simulink model "objectDetector"  (R2016b)
settings: Solver=FixedStepAuto  StartTime=0.0  StopTime=inf  RelTol=1e-3
model workspace (MAT data in the model file):
  SL_ROS_VariableLengthArrays_MaxSizes.CommonInfo.ArrayTruncateAction = 'EmitWarning'
  SL_ROS_VariableLengthArrays_MaxSizes.MsgTypeMap = containers.Map
  SL_ROS_VariableLengthArrays_MaxSizes.MsgTypeMap.serialization.keys = {'sensor_msgs/LaserScan'}
  SL_ROS_VariableLengthArrays_MaxSizes.MsgTypeMap.serialization.values{1}(1).PropertyName = 'Ranges'
  SL_ROS_VariableLengthArrays_MaxSizes.MsgTypeMap.serialization.values{1}(1).DataType = 'single'
  SL_ROS_VariableLengthArrays_MaxSizes.MsgTypeMap.serialization.values{1}(1).MaxLength = 180
  SL_ROS_VariableLengthArrays_MaxSizes.MsgTypeMap.serialization.values{1}(2).PropertyName = 'Intensities'
  SL_ROS_VariableLengthArrays_MaxSizes.MsgTypeMap.serialization.values{1}(2).DataType = 'single'
  SL_ROS_VariableLengthArrays_MaxSizes.MsgTypeMap.serialization.values{1}(2).MaxLength = 128
  SL_ROS_VariableLengthArrays_MaxSizes.MsgTypeMap.serialization.uniformity = 0
  SL_ROS_VariableLengthArrays_MaxSizes.MsgTypeMap.serialization.keyType = 'char'
  SL_ROS_VariableLengthArrays_MaxSizes.MsgTypeMap.serialization.valueType = 'any'
undefined symbols (not defined in the file): Header
libraries: robotlib x4
settings Model: Creator=jupan  LastModifiedBy=fred
settings SolverCC: AutoInsertRateTranBlk=on
settings OptimizationCC: MaxStackSize=64
settings DebuggingCC: ParameterTunabilityLossMsg=error
settings HardwareCC: ProdBitPerPointer=32  ProdBitPerSizeT=32  ProdBitPerPtrDiffT=32  ProdLargestAtomicFloat=None  ProdIntDivRoundTo=Undefined  ProdEndianess=Unspecified  ProdWordSize=32  ProdHWDeviceType=Generic->Unspecified (assume 32-bit Generic)
settings RTWCC: SystemTargetFile=ert.tlc  HardwareBoard=Robot Operating System (ROS)  TLCOptions="-aInlineSetEventsForThisBaseRateFcn=TLC_FALSE -aSuppressMultiTaskScheduler=TLC_FALSE  -aRateBasedStepFcn=0"  TemplateMakefile=ert_default_tmf  Description=Embedded Coder  GenerateReport=on  Toolchain=Catkin  IncludeHyperlinkInReport=on  LaunchReport=on  TargetLang=C++  GenerateTraceInfo=on  GenerateTraceReport=on  GenerateTraceReportSl=on  GenerateTraceReportSf=on  GenerateTraceReportEml=on
settings CodeAppCC: ForceParamTrailComments=on  IgnoreCustomStorageClasses=off  OperatorAnnotations=on  SimulinkDataObjDesc=on  SFDataObjDesc=on  MATLABFcnDesc=on  InsertBlockDesc=on  MATLABSourceComments=on
settings ERTTargetCC: SupportVariableSizeSignals=on

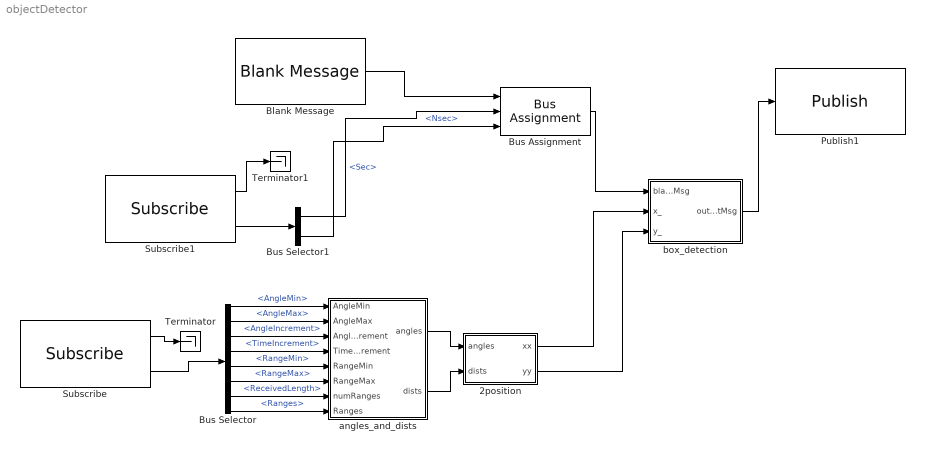
== system objectDetector ==
  " 2position" : MATLAB Function  TreatAsAtomicUnit=on
  Blank Message : robotlib/Blank Message  SourceLibraryInfo=This block requires Robotics System Toolbox  messageType=geometry_msgs/PolygonStamped  SampleTime=inf
  Bus Assignment : BusAssignment  AssignedSignals=Header.Stamp.Sec,Header.Stamp.Nsec
  Bus Selector : BusSelector  OutputSignals=AngleMin,AngleMax,AngleIncrement,TimeIncrement,RangeMin,RangeMax,Ranges_SL_Info.ReceivedLength,Ranges
  Bus Selector1 : BusSelector  OutputSignals=Clock_.Sec,Clock_.Nsec
  Publish1 : robotlib/Publish  SourceLibraryInfo=This block requires Robotics System Toolbox  topicSource=Specify your own  topic=/detections  messageType=geometry_msgs/PolygonStamped  messageQueueLength=1
  Subscribe : robotlib/Subscribe  SourceLibraryInfo=This block requires Robotics System Toolbox  topicSource=Select from ROS network  topic=/catvehicle/front_laser_points  messageType=sensor_msgs/LaserScan  sampleTime=-1  messageQueueLength=1
  Subscribe1 : robotlib/Subscribe  SourceLibraryInfo=This block requires Robotics System Toolbox  topicSource=Select from ROS network  topic=/clock  messageType=rosgraph_msgs/Clock  sampleTime=-1  messageQueueLength=1
  Terminator : Terminator
  Terminator1 : Terminator
  angles_and_dists : MATLAB Function  TreatAsAtomicUnit=on
  box_detection : MATLAB Function  TreatAsAtomicUnit=on
  wires:
  Subscribe/1 -> Terminator/1
  Subscribe/2 -> Bus Selector/1
  Bus Selector/1 -> angles_and_dists/1(AngleMin)  "<AngleMin>"
  Bus Selector/2 -> angles_and_dists/2(AngleMax)  "<AngleMax>"
  Bus Selector/3 -> angles_and_dists/3(AngleIncrement)  "<AngleIncrement>"
  Bus Selector/4 -> angles_and_dists/4(TimeIncrement)  "<TimeIncrement>"
  Bus Selector/5 -> angles_and_dists/5(RangeMin)  "<RangeMin>"
  Bus Selector/6 -> angles_and_dists/6(RangeMax)  "<RangeMax>"
  Bus Selector/7 -> angles_and_dists/7(numRanges)  "<ReceivedLength>"
  Bus Selector/8 -> angles_and_dists/8(Ranges)  "<Ranges>"
  Blank Message/1 -> Bus Assignment/1
  box_detection/1(outputMsg) -> Publish1/1
  Bus Assignment/1 -> box_detection/1(blankMsg)
  Subscribe1/1 -> Terminator1/1
  Subscribe1/2 -> Bus Selector1/1
  Bus Selector1/1 -> Bus Assignment/2  "<Sec>"
  Bus Selector1/2 -> Bus Assignment/3  "<Nsec>"
  angles_and_dists/1(angles) -> " 2position"/1(angles)
  angles_and_dists/2(dists) -> " 2position"/2(dists)
  " 2position"/1(xx) -> box_detection/2(x_)
  " 2position"/2(yy) -> box_detection/3(y_)

== matlab function objectDetector/ 2position ==
  data: angles input size=[180 1]; xx output size=[180 1]; dists input size=[180 1]; yy output size=[180 1]
function [xx, yy] = fcn(angles, dists)

%#codegen
xx = dists.*cos(angles);
yy = dists.*sin(angles);
% flag = 1;
% tmp = 0;
% for i = 1 : 180
%     if(xx(i) ~= 0 && flag == 1)
%         tmp = i;
%         flag = 0;
%     elseif(xx(i) == 0)
%         flag = 1;
%     else
%         xx(tmp) = (xx(tmp) + xx(i))/2;
%         yy(tmp) = (yy(tmp) + yy(i))/2;
%         xx(i) = 0;
%         yy(i) = 0;
%     end 
% end

== matlab function objectDetector/angles_and_dists ==
  data: AngleMin input size=1; angles output size=[180 1]; dists output size=[180 1]; AngleMax input; AngleIncrement input; TimeIncrement input; RangeMin input; RangeMax input; numRanges input; Ranges input
function [angles,dists] = fcn(AngleMin, AngleMax, AngleIncrement, ...
                TimeIncrement, RangeMin, RangeMax, numRanges, Ranges )
%#codegen

% this function transforms the laser scan into cartesian coordinates, so
% that you can use other tools to group them together, make an image, etc.
angleMin = AngleMin;
angleMax = AngleMax;
angleIncrement = AngleIncrement;
timeIncrement = TimeIncrement;
rangeMin = RangeMin;
rangeMax = RangeMax;
ranges = Ranges;
ranges(ranges>RangeMax) = NaN;
ranges(ranges<RangeMin) = NaN;
%rangesLength = scan.Ranges_SL_Info.ReceivedLength;
%intensities = scan.Intensities;
flag = 1;
dists = zeros(180, 1);
% for i = 1:180
%     if(ranges(i) == 80)
%         dists(i) = 0;
%     else
%         dists(i) = ranges(i)+2;
%     end
% end
tmp = 0;
for i = 1 : 180
    if(ranges(i) ~= 80.0 && flag == 1)
        dists(i) = ranges(i);
        tmp = i;
        flag = 0;
    elseif(ranges(i) == 80.0)
        flag = 1;
        dists(i) = 0;
    else
        dists(tmp) = (dists(tmp) + ranges(i))/2;
        dists(i) = 0;
    end 
end
angles = [-pi/2:pi/179:pi/2]';
%dists = [tmp];

== matlab function objectDetector/box_detection ==
  data: blankMsg input; x_ input; outputMsg output SL_Bus_objectDetector_geometry_msgs_PolygonStamped; y_ input
    function outputMsg = fcn(blankMsg, x_, y_)
    %#codegen
    % the sequence of the message must increment each time we publish, so we
    % need it to be persistent across instantiations
    xc = zeros(180, 1);
    yc = zeros(180, 1);
    k = 1;
    for i = 1:180
        if(x_(i) ~= 0)
            xc(k) = x_(i);
            yc(k) = y_(i);
            k = k + 1;
        end
    end
    xk = zeros(k, 1);
    yk = zeros(k, 1);
    for j = 1:k
        xk(j) = xc(j);
        yk(j) = yc(j);
    end
    
    persistent seq;

    % if this is the first time our model is run, then 'seq' will not exist.
    % Then 'isempty(seq)' will be true, which allows us to intialize it to 0
    if isempty(seq)
        seq=uint32(0);
    end

    % increment the sequence number
    seq = seq+1;
    % set our output to be a copy of the input (blankMsg)
    outputMsg = blankMsg;
    % these points in (x,y,z) are either taken from the inputs, or hardcoded
    z = single(0);
    % by definition in this block, we are making a square.
    % IF YOU USE THIS model as inspiration for an output detection that is a
    % pentagon, then you would set the length to be 5, for example.
    outputMsg.Polygon.Points_SL_Info.CurrentLength = uint32(4);
    % set the frame to be relative to our base of 0. If you want to use data
    % coming from another detection, then you can set the /detections to be in
    % the frame of that specific sensor
    str = 'catvehicle/odom';
    % initialize the header and set its values
    strLength = length(str);
    outputMsg.Header.Seq = seq;
    outputMsg.Header.FrameId(1:strLength) = str;
    outputMsg.Header.FrameId_SL_Info.CurrentLength = uint32(strLength);
    if(mod(seq,k) ~= 0)
        id = mod(seq,k);
    else
        id = uint32(k);
    end
    if(yk(id) < 0)
        xtmp = xk(id) + 2;
        ytmp = yk(id) + 2;
    elseif(yk(id) < 1 && yk(id) > 0)
        xtmp = xk(id) + 1;
        ytmp = yk(id);
    else
        xtmp = xk(id)+1;
        ytmp = yk(id)+1;
    end
    % populate point 1
    outputMsg.Polygon.Points(1).X = floor(single(xtmp));
    outputMsg.Polygon.Points(1).Y = floor(single(ytmp));
    outputMsg.Polygon.Points(1).Z = z;

    % populate point 2
    outputMsg.Polygon.Points(2).X = floor(single(xtmp));
    outputMsg.Polygon.Points(2).Y = ceil(single(ytmp));
    outputMsg.Polygon.Points(2).Z = z;

    % populate point 3
    outputMsg.Polygon.Points(3).X = ceil(single(xtmp));
    outputMsg.Polygon.Points(3).Y = ceil(single(ytmp));
    outputMsg.Polygon.Points(3).Z = z;

    % populate point 4
    outputMsg.Polygon.Points(4).X = ceil(single(xtmp));
    outputMsg.Polygon.Points(4).Y = floor(single(ytmp));
    outputMsg.Polygon.Points(4).Z = z;
    
        
    end
    
    
    
   
    % note that the polygon type "closes" between the last and first points
